simulink model "navigation_filter_flat_earth_noise"  (R2024a)
settings: Solver=VariableStepAuto  StartTime=0.0  StopTime=time(end)  RelTol=1e-3
values from neighbouring files (symbols this model uses):
  pos = pos_f    [test_traj_gen_v2 1.m]    (also in test_traj_gen_v2.m)
  rpy = zeros(length(time),3)    [test_traj_gen_v2 1.m]    (also in test_traj_gen_v2.m)
  ST = 1/100    (= 0.01)    [test_traj_gen_v2 1.m]    (also in test_traj_gen_v2.m)
  vel_n = vel_n_f    [test_traj_gen_v2 1.m]    (also in test_traj_gen_v2.m)
undefined symbols (not defined in the file or in its folder): DiscIntNeverNeededParam
libraries: simulink x8, cstblocks x3
settings Model: Creator=Lorenzo  LastModifiedBy=Lorenzo
settings RTWCC: GPUComputeCapability=3.5

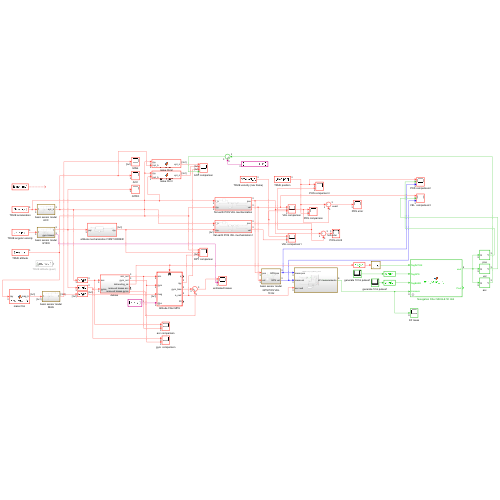
[thumbnail: Simulink's stored preview of the top-level diagram]
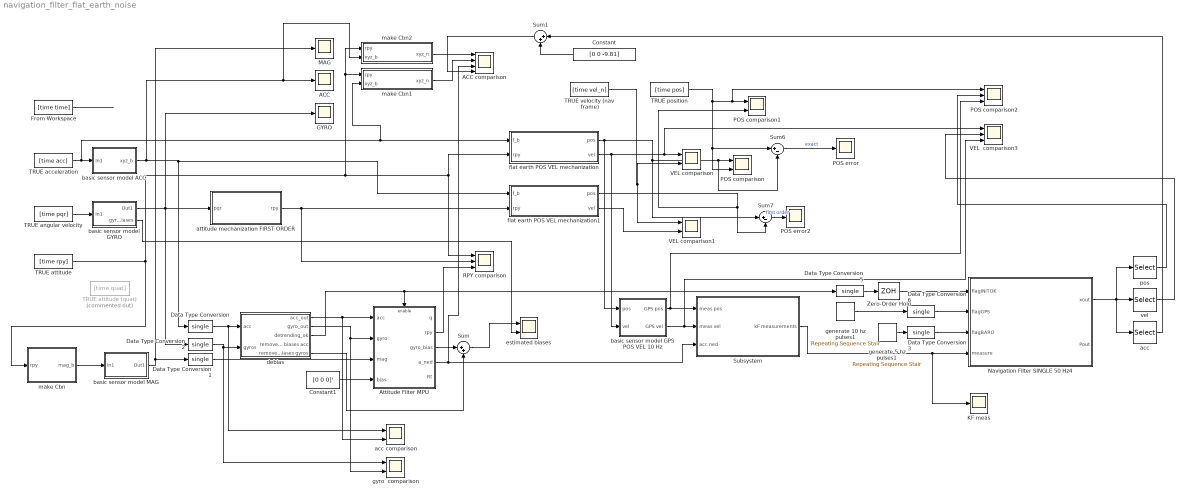
== system navigation_filter_flat_earth_noise ==
  ACC : Scope
  ACC comparison : Scope  NumInputPorts=4
  Attitude Filter MPU : Subsystem  mask{T=ST}
      mask prompts: T "Sample Time"
  Constant : Constant  Value=[0 0 -9.81]
  Constant1 : Constant  Value=[0 0 0]'  OutDataTypeStr=single
  Data Type Conversion{,1..3,5..6} (6 alike) : DataTypeConversion  OutDataTypeStr=single  SaturateOnIntegerOverflow=off  RndMeth=Floor
  From Workspace : FromWorkspace  VariableName=[time time]  SampleTime=ST
  GYRO : Scope
  KF meas : Scope
  MAG : Scope
  "Navigation Filter SINGLE 50 Hz4 " : MATLAB Function  TreatAsAtomicUnit=on  mask{Q=single(diag([1e-8, 1e-4, 1e-2, 1e-8, 1e-4, 1e-2, 1e-5, 1e-4, 0.010]))*2, GPS_cov=single([0.1, 0.1, 10, 10, 0.36])/2, IMU_cov=single([15*[0.07, 0.07] 10*0.09])/2, BARO_cov=single(1.7)/2}
      mask prompts: Q "Q matrix"; GPS_cov "R matrix - GPS covariance [px py vx vy vz]"; IMU_cov "R matrix - IMU covariance [ax ay az]"; BARO_cov "R matrix - BARO covariance"
  POS comparison : Scope  NumInputPorts=2
  POS comparison1 : Scope  NumInputPorts=2
  POS comparison2 : Scope  NumInputPorts=3
  POS error : Scope
  POS error2 : Scope
  RPY comparison : Scope  NumInputPorts=3
  Subsystem : Subsystem
  Sum : Sum  Inputs=|++
  Sum1 : Sum  Inputs=|++
  Sum6 : Sum  Inputs=|+-
  Sum7 : Sum  Inputs=|+-
  TRUE acceleration : FromWorkspace  VariableName=[time acc]  SampleTime=ST
  TRUE angular velocity : FromWorkspace  VariableName=[time pqr]  SampleTime=ST
  TRUE attitude : FromWorkspace  VariableName=[time rpy]  SampleTime=ST
  TRUE attitude (quat) : FromWorkspace  Commented=on  VariableName=[time quat]
  TRUE position : FromWorkspace  VariableName=[time pos]  SampleTime=ST
  TRUE velocity (nav frame) : FromWorkspace  VariableName=[time vel_n]  SampleTime=ST
  VEL  comparison3 : Scope  NumInputPorts=3
  VEL comparison : Scope  NumInputPorts=2
  VEL comparison1 : Scope  NumInputPorts=2
  Zero-Order Hold : ZeroOrderHold  SampleTime=0.02
  acc : Selector  InputPortWidth=9  IndexOptions=Index vector (dialog)  Indices=[1 4 7]+2  OutputSizes=1
  acc comparison : Scope  NumInputPorts=2
  attitude mechanization FIRST ORDER : Subsystem
  basic sensor model ACC : Subsystem
  basic sensor model GPS POS VEL 10 Hz : Subsystem
  basic sensor model GYRO : Subsystem
  basic sensor model MAG : Subsystem
  "debias " : Subsystem
  estimated biases : Scope  NumInputPorts=2
  flat earth POS VEL mechanization : Subsystem
  flat earth POS VEL mechanization1 : Subsystem
  generate 10 hz pulses1 : simulink/Sources/Repeating Sequence Stair  OutValues=[ 0 0 0 0 1].'  tsamp=1/50  OutMin=[]  OutMax=[]  OutDataTypeStr=double  OutputDataTypeScalingMode=double  OutDataType=fixdt(0,8)  ConRadixGroup=Best Precision: Vector-wise  OutScaling=2^-12
  generate 5 hz pulses1 : simulink/Sources/Repeating Sequence Stair  OutValues=[ 0 0 0 0 0 0 0 0 1].'  tsamp=1/50  OutMin=[]  OutMax=[]  OutDataTypeStr=double  OutputDataTypeScalingMode=double  OutDataType=fixdt(0,8)  ConRadixGroup=Best Precision: Vector-wise  OutScaling=2^-12
  gyro  comparison : Scope  NumInputPorts=2
  make Cbn : MATLAB Function  TreatAsAtomicUnit=on
  make Cbn1 : MATLAB Function  TreatAsAtomicUnit=on
  make Cbn2 : MATLAB Function  TreatAsAtomicUnit=on
  pos : Selector  InputPortWidth=9  IndexOptions=Index vector (dialog)  Indices=[1 4 7]  OutputSizes=1
  vel : Selector  InputPortWidth=9  IndexOptions=Index vector (dialog)  Indices=[1 4 7]+1  OutputSizes=1
  wires:
  From Workspace/1 -> ?
  TRUE position/1 -> POS comparison2/1, POS comparison1/1, Sum6/1, POS comparison/2
  TRUE velocity (nav frame)/1 -> VEL comparison1/1, VEL comparison/2
  flat earth POS VEL mechanization/1(pos) -> basic sensor model GPS POS VEL 10 Hz/1(pos), Sum7/1, Sum6/2, POS comparison/1
  flat earth POS VEL mechanization/2(vel) -> basic sensor model GPS POS VEL 10 Hz/2(vel), VEL  comparison3/1, VEL comparison/1
  TRUE angular velocity/1 -> basic sensor model GYRO/1(In1)
  attitude mechanization FIRST ORDER/1(rpy) -> RPY comparison/2, flat earth POS VEL mechanization1/2(rpy)
  TRUE attitude/1 -> make Cbn/1(rpy), make Cbn1/1(rpy), make Cbn2/1(rpy), RPY comparison/1, flat earth POS VEL mechanization/2(rpy)
  Sum6/1 -> POS error/1  "exact"
  Sum7/1 -> POS error2/1  "first order"
  flat earth POS VEL mechanization1/1(pos) -> Sum7/2, POS comparison1/2
  basic sensor model ACC/1(xyz_b) -> make Cbn2/2(xyz_b), ACC/1, Data Type Conversion/1, flat earth POS VEL mechanization1/1(f_b)
  TRUE acceleration/1 -> make Cbn1/2(xyz_b), flat earth POS VEL mechanization/1(f_b), basic sensor model ACC/1(In1)
  basic sensor model GYRO/1(Out1) -> attitude mechanization FIRST ORDER/1(pqr), Data Type Conversion2/1, GYRO/1
  flat earth POS VEL mechanization1/2(vel) -> VEL comparison1/2
  make Cbn/1(mag_b) -> basic sensor model MAG/1(In1)
  basic sensor model MAG/1(Out1) -> MAG/1, Data Type Conversion1/1
  Constant1/1 -> Attitude Filter MPU/4(bias)
  Attitude Filter MPU/2(rpy) -> RPY comparison/3
  Data Type Conversion/1 -> acc comparison/1, "debias "/1(acc)
  Data Type Conversion2/1 -> gyro  comparison/1, "debias "/2(gyros)
  Attitude Filter MPU/3(gyro_bias) -> Sum/1
  basic sensor model GYRO/2(gyro biases) -> estimated biases/2
  "debias "/3(detrending_ok) -> Attitude Filter MPU/Enable, Data Type Conversion5/1
  "debias "/1(acc_out) -> acc comparison/2, Attitude Filter MPU/1(acc)
  "debias "/2(gyro_out) -> gyro  comparison/2, Attitude Filter MPU/2(gyro)
  Data Type Conversion1/1 -> Attitude Filter MPU/3(mag)
  "debias "/5(removed biases gyros) -> Sum/2
  Sum/1 -> estimated biases/1
  basic sensor model GPS POS VEL 10 Hz/1("GPS pos ") -> POS comparison2/3, Subsystem/1("meas pos ")
  "Navigation Filter SINGLE 50 Hz4 "/1(xout) -> acc/1, vel/1, pos/1
  pos/1 -> POS comparison2/2
  vel/1 -> VEL  comparison3/2
  basic sensor model GPS POS VEL 10 Hz/2(GPS vel) -> VEL  comparison3/3, Subsystem/2(meas vel)
  acc/1 -> Sum1/1
  Attitude Filter MPU/4(a_ned) -> Subsystem/3(acc ned), ACC comparison/3
  Subsystem/1(kF measurements) -> KF meas/1, "Navigation Filter SINGLE 50 Hz4 "/4(measure)
  generate 10 hz pulses1/1 -> Data Type Conversion6/1
  generate 5 hz pulses1/1 -> Data Type Conversion3/1
  Data Type Conversion6/1 -> "Navigation Filter SINGLE 50 Hz4 "/2(flagGPS)
  Data Type Conversion3/1 -> "Navigation Filter SINGLE 50 Hz4 "/3(flagBARO)
  Data Type Conversion5/1 -> Zero-Order Hold/1
  make Cbn1/1(xyz_n) -> ACC comparison/2
  make Cbn2/1(xyz_n) -> ACC comparison/1
  Sum1/1 -> ACC comparison/4
  Constant/1 -> Sum1/2
  Zero-Order Hold/1 -> "Navigation Filter SINGLE 50 Hz4 "/1(flagINITOK)

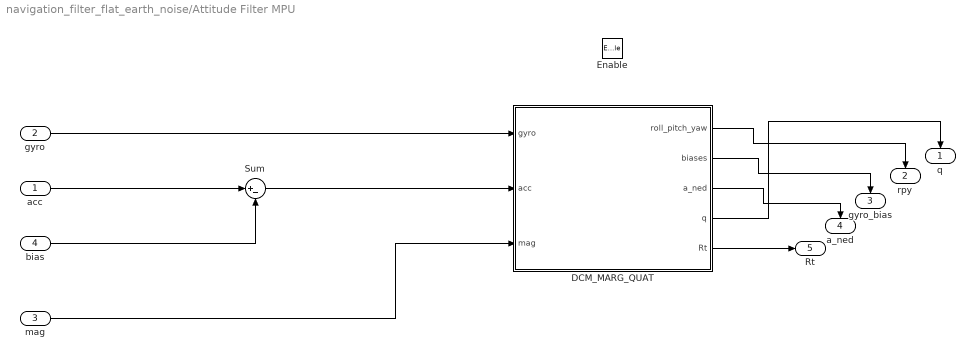
== system navigation_filter_flat_earth_noise/Attitude Filter MPU ==
  acc : Inport
  gyro : Inport  Port=2
  mag : Inport  Port=3
  bias : Inport  Port=4
  Enable : EnablePort  StatesWhenEnabling=reset
  DCM_MARG_QUAT : Subsystem  mask{Kp=0.15, Ki=0.005, tau=40, T=T}
      mask prompts: Kp "Proportional Gain"; Ki "Integral Gain"; tau "Biases Time Constant"; T "Sample Time"
  Sum : Sum  Inputs=|+-
  q : Outport  PortDimensions=4  InitialOutput=[1 0 0 0]'
  rpy : Outport  Port=2  PortDimensions=3  InitialOutput=[0 0 0]'
  gyro_bias : Outport  Port=3  PortDimensions=3  InitialOutput=[0 0 0]'
  a_ned : Outport  Port=4  InitialOutput=[0 0 0]'
  Rt : Outport  Port=5
  wires:
  mag/1 -> DCM_MARG_QUAT/3(mag)
  DCM_MARG_QUAT/4(q) -> q/1
  bias/1 -> Sum/2
  Sum/1 -> DCM_MARG_QUAT/2(acc)
  acc/1 -> Sum/1
  DCM_MARG_QUAT/3(a_ned) -> a_ned/1
  DCM_MARG_QUAT/1(roll_pitch_yaw) -> rpy/1
  gyro/1 -> DCM_MARG_QUAT/1(gyro)
  DCM_MARG_QUAT/2(biases) -> gyro_bias/1
  DCM_MARG_QUAT/5(Rt) -> Rt/1

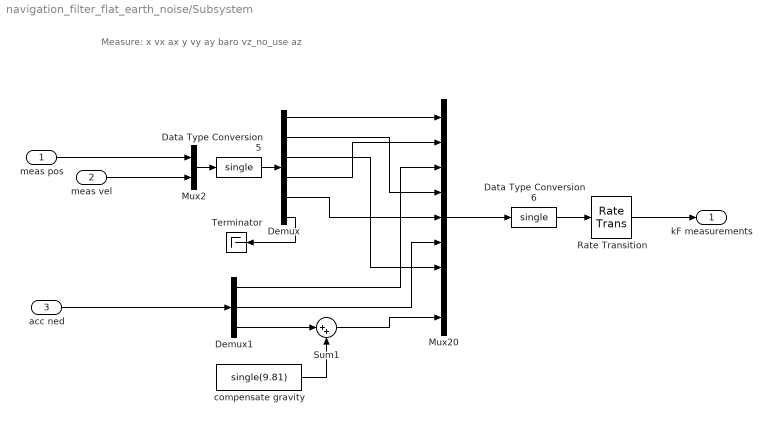
== system navigation_filter_flat_earth_noise/Subsystem ==
  note: Measure: x vx ax y vy ay baro vz_no_use az
  "meas pos " : Inport
  meas vel : Inport  Port=2
  acc ned : Inport  Port=3
  Data Type Conversion5 : DataTypeConversion  OutDataTypeStr=single  SaturateOnIntegerOverflow=off  RndMeth=Floor
  Data Type Conversion6 : DataTypeConversion  OutDataTypeStr=single  SaturateOnIntegerOverflow=off  RndMeth=Floor
  Demux : Demux  Outputs=6
  Demux1 : Demux  Outputs=3
  Mux2 : Mux  Inputs=2
  Mux20 : Mux  Inputs=9
  Rate Transition : RateTransition  OutPortSampleTime=1/50
  Sum1 : Sum  Inputs=|++
  Terminator : Terminator
  compensate gravity : Constant  Value=single(9.81)
  kF measurements : Outport
  wires:
  Demux/5 -> Mux20/5
  Sum1/1 -> Mux20/9
  Demux/4 -> Mux20/2
  Mux20/1 -> Data Type Conversion6/1
  Demux1/3 -> Sum1/1
  Data Type Conversion5/1 -> Demux/1
  Demux/6 -> Terminator/1
  Demux/1 -> Mux20/1
  ? -> Mux20/8
  Data Type Conversion6/1 -> Rate Transition/1
  Mux2/1 -> Data Type Conversion5/1
  Demux1/2 -> Mux20/6
  "meas pos "/1 -> Mux2/1
  compensate gravity/1 -> Sum1/2
  Demux/3 -> Mux20/7
  Demux1/1 -> Mux20/3
  Demux/2 -> Mux20/4
  meas vel/1 -> Mux2/2
  acc ned/1 -> Demux1/1
  Rate Transition/1 -> kF measurements/1

== system navigation_filter_flat_earth_noise/attitude mechanization FIRST ORDER ==
  pqr : Inport
  Attitude Mechanization : MATLAB Function  TreatAsAtomicUnit=on
  rpy_mem : UnitDelay  InitialCondition=rpy(1,:)'  SampleTime=-1  HasFrameUpgradeWarning=on
  rpy : Outport
  wires:
  pqr/1 -> Attitude Mechanization/1(pqr)
  rpy_mem/1 -> Attitude Mechanization/2(rpy_)
  Attitude Mechanization/1(rpy) -> rpy_mem/1, rpy/1

== system navigation_filter_flat_earth_noise/basic sensor model ACC ==
  note: [0.05 0.1 0.15]
  In1 : Inport
  Add : Sum  Inputs=+++
  Mux : Mux  Inputs=2
  Scope : Scope
  White Noise acc : RandomNumber  DisableCoverage=on  Mean=[0 0 0 ]  Variance=[0.006 0.006 0.006].^2  Seed=[1 2 3]  SampleTime=1/50
  bias : Constant  Value=[0.05 0.1 0.15]
  xyz_b : Outport
  wires:
  In1/1 -> Mux/2, Add/1
  White Noise acc/1 -> Add/3
  bias/1 -> Add/2
  Mux/1 -> Scope/1
  Add/1 -> Mux/1, xyz_b/1

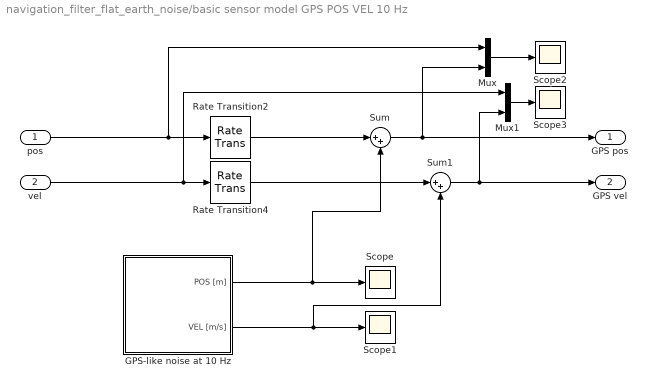
== system navigation_filter_flat_earth_noise/basic sensor model GPS POS VEL 10 Hz ==
  pos : Inport
  vel : Inport  Port=2
  GPS-like noise at 10 Hz : Subsystem  mask{AMPX=3, AMPY=3, AMPZ=0.5, newnoise=off, seed_user=0}
      mask prompts: AMPX "gps approx max error X [m]"; AMPY "gps approx max error Y [m]"; AMPZ "gps approx max error Z [m]"; newnoise "new noise at each run"; seed_user "user provided seed value"
      mask init:
      | if newnoise,
      |         seedx=rand(1)*1000;
      |         seedy=rand(1)*1000;
      |         seedz=rand(1)*1000;
      |     else
      |         seedx=seed_user;
      |         seedy=seed_user+1;
      |         seedz=seed_user+2;
      |     end
      mask DialogControl ParameterGroupVar Prompt: Noise generation
  Mux : Mux  Inputs=2
  Mux1 : Mux  Inputs=2
  Rate Transition2 : RateTransition  OutPortSampleTime=1/10
  Rate Transition4 : RateTransition  OutPortSampleTime=1/10
  Scope{,1..3} (4 alike) : Scope
  Sum : Sum  Inputs=|++
  Sum1 : Sum  Inputs=|++
  "GPS pos " : Outport
  GPS vel : Outport  Port=2
  wires:
  pos/1 -> Mux/1, Rate Transition2/1
  vel/1 -> Mux1/1, Rate Transition4/1
  GPS-like noise at 10 Hz/2(VEL [m/s]) -> Sum1/2, Scope1/1
  GPS-like noise at 10 Hz/1(POS [m]) -> Sum/2, Scope/1
  Mux/1 -> Scope2/1
  Sum/1 -> "GPS pos "/1, Mux/2
  Sum1/1 -> Mux1/2, GPS vel/1
  Rate Transition2/1 -> Sum/1
  Rate Transition4/1 -> Sum1/1
  Mux1/1 -> Scope3/1

== system navigation_filter_flat_earth_noise/basic sensor model GYRO ==
  In1 : Inport
  Add : Sum  Inputs=+++
  Mux : Mux  Inputs=2
  Scope : Scope
  White Noise gyro : RandomNumber  DisableCoverage=on  Mean=[0 0 0]  Variance=[0.003 0.003 0.003].^2  Seed=[4 5 6]  SampleTime=1/50
  bias : Constant  Value=[0.03 0.06 0.09]
  Out1 : Outport
  gyro biases : Outport  Port=2
  wires:
  White Noise gyro/1 -> Add/3
  bias/1 -> Add/2, gyro biases/1
  Mux/1 -> Scope/1
  In1/1 -> Mux/2, Add/1
  Add/1 -> Mux/1, Out1/1

== system navigation_filter_flat_earth_noise/basic sensor model MAG ==
  In1 : Inport
  Add : Sum  Inputs=+++
  Mux : Mux  Inputs=2
  Scope : Scope
  White Noise mag : RandomNumber  DisableCoverage=on  Mean=[0 0 0]  Variance=[0.003 0.003 0.003].^2  Seed=[7 8 9]  SampleTime=1/50
  bias : Constant  Value=[0.0 0.0 0.0]
  Out1 : Outport
  wires:
  Add/1 -> Out1/1, Mux/1
  In1/1 -> Add/1, Mux/2
  Mux/1 -> Scope/1
  bias/1 -> Add/2
  White Noise mag/1 -> Add/3

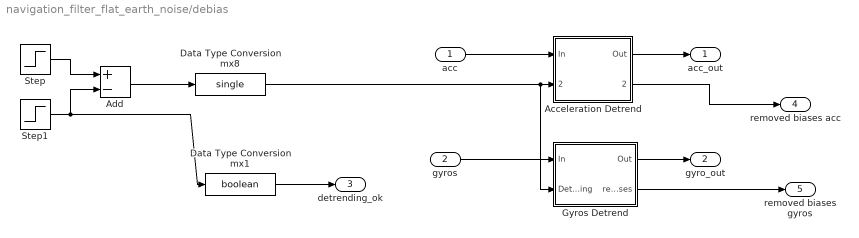
== system navigation_filter_flat_earth_noise/debias  ==
  acc : Inport
  gyros : Inport  Port=2
  "Acceleration Detrend " : Subsystem  mask{ST2=ST}
      mask prompts: ST2 "Sample Time"
  Add : Sum  Inputs=+-
  Data Type Conversion mx1 : DataTypeConversion  OutDataTypeStr=boolean  RndMeth=Round
  Data Type Conversion mx8 : DataTypeConversion  OutDataTypeStr=single  RndMeth=Round
  Gyros Detrend : Subsystem  mask{ST2=ST}
      mask prompts: ST2 "Sample Time"
  Step : Step  Time=0.1  SampleTime=ST
  Step1 : Step  SampleTime=ST
  acc_out : Outport
  gyro_out : Outport  Port=2
  detrending_ok : Outport  Port=3
  removed biases acc : Outport  Port=4
  removed biases gyros : Outport  Port=5
  wires:
  Step/1 -> Add/1
  Step1/1 -> Add/2, Data Type Conversion mx1/1
  Add/1 -> Data Type Conversion mx8/1
  acc/1 -> "Acceleration Detrend "/1(In)
  gyros/1 -> Gyros Detrend/1(In)
  "Acceleration Detrend "/1(Out) -> acc_out/1
  Gyros Detrend/1(Out) -> gyro_out/1
  Data Type Conversion mx1/1 -> detrending_ok/1
  Data Type Conversion mx8/1 -> Gyros Detrend/2(Detrending), "Acceleration Detrend "/2(Detrending)
  "Acceleration Detrend "/2(removed biases) -> removed biases acc/1
  Gyros Detrend/2(removed biases) -> removed biases gyros/1

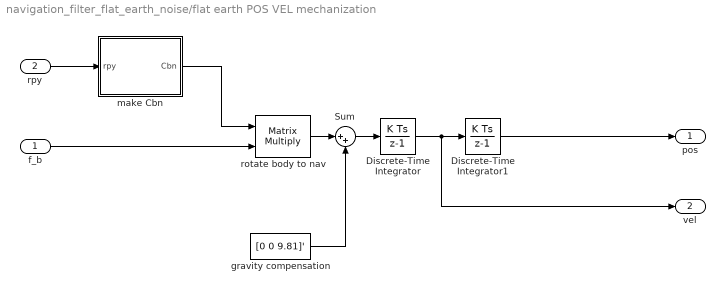
== system navigation_filter_flat_earth_noise/flat earth POS VEL mechanization ==
  f_b : Inport
  rpy : Inport  Port=2
  Discrete-Time Integrator : DiscreteIntegrator  InitialCondition=vel_n(1,:)  SampleTime=-1  ICPrevOutput=DiscIntNeverNeededParam  ICPrevScaledInput=DiscIntNeverNeededParam
  Discrete-Time Integrator1 : DiscreteIntegrator  InitialCondition=pos(1,:)  SampleTime=-1  ICPrevOutput=DiscIntNeverNeededParam  ICPrevScaledInput=DiscIntNeverNeededParam
  Sum : Sum  Inputs=|++
  gravity compensation : Constant  Value=[0 0 9.81]'
  make Cbn : MATLAB Function  TreatAsAtomicUnit=on
  rotate body to nav : Product  Multiplication=Matrix(*)
  pos : Outport
  vel : Outport  Port=2
  wires:
  rotate body to nav/1 -> Sum/1
  gravity compensation/1 -> Sum/2
  Discrete-Time Integrator/1 -> vel/1, Discrete-Time Integrator1/1
  make Cbn/1(Cbn) -> rotate body to nav/1
  Discrete-Time Integrator1/1 -> pos/1
  Sum/1 -> Discrete-Time Integrator/1
  f_b/1 -> rotate body to nav/2
  rpy/1 -> make Cbn/1(rpy)

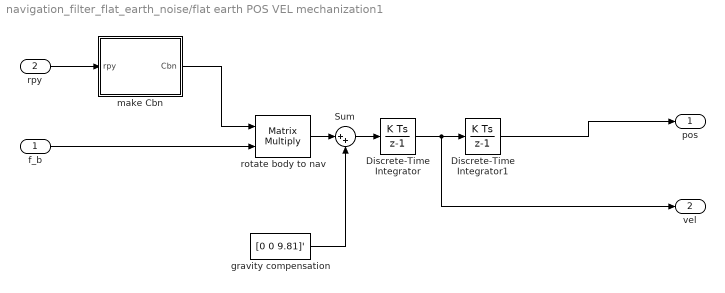
== system navigation_filter_flat_earth_noise/flat earth POS VEL mechanization1 ==
  f_b : Inport
  rpy : Inport  Port=2
  Discrete-Time Integrator : DiscreteIntegrator  InitialCondition=vel_n(1,:)  SampleTime=-1  ICPrevOutput=DiscIntNeverNeededParam  ICPrevScaledInput=DiscIntNeverNeededParam
  Discrete-Time Integrator1 : DiscreteIntegrator  InitialCondition=pos(1,:)  SampleTime=-1  ICPrevOutput=DiscIntNeverNeededParam  ICPrevScaledInput=DiscIntNeverNeededParam
  Sum : Sum  Inputs=|++
  gravity compensation : Constant  Value=[0 0 9.81]'
  make Cbn : MATLAB Function  TreatAsAtomicUnit=on
  rotate body to nav : Product  Multiplication=Matrix(*)
  pos : Outport
  vel : Outport  Port=2
  wires:
  rpy/1 -> make Cbn/1(rpy)
  f_b/1 -> rotate body to nav/2
  Sum/1 -> Discrete-Time Integrator/1
  Discrete-Time Integrator1/1 -> pos/1
  make Cbn/1(Cbn) -> rotate body to nav/1
  Discrete-Time Integrator/1 -> Discrete-Time Integrator1/1, vel/1
  gravity compensation/1 -> Sum/2
  rotate body to nav/1 -> Sum/1

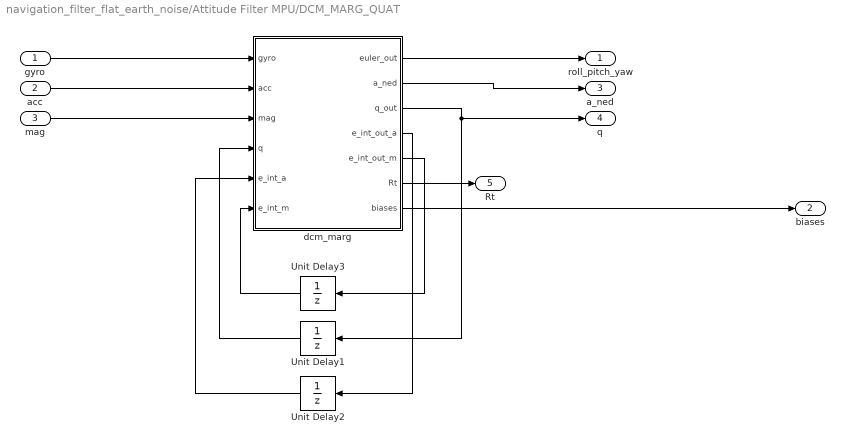
== system navigation_filter_flat_earth_noise/Attitude Filter MPU/DCM_MARG_QUAT ==
  gyro : Inport
  acc : Inport  Port=2
  mag : Inport  Port=3
  Unit Delay1 : UnitDelay  InitialCondition=[1;0;0;0]  SampleTime=T  HasFrameUpgradeWarning=on
  Unit Delay2 : UnitDelay  SampleTime=T  HasFrameUpgradeWarning=on
  Unit Delay3 : UnitDelay  SampleTime=T  HasFrameUpgradeWarning=on
  dcm_marg : MATLAB Function  TreatAsAtomicUnit=on
  roll_pitch_yaw : Outport
  biases : Outport  Port=2
  a_ned : Outport  Port=3
  q : Outport  Port=4
  Rt : Outport  Port=5
  wires:
  Unit Delay3/1 -> dcm_marg/6(e_int_m)
  dcm_marg/5(e_int_out_m) -> Unit Delay3/1
  dcm_marg/2(a_ned) -> a_ned/1
  dcm_marg/1(euler_out) -> roll_pitch_yaw/1
  gyro/1 -> dcm_marg/1(gyro)
  acc/1 -> dcm_marg/2(acc)
  mag/1 -> dcm_marg/3(mag)
  dcm_marg/3(q_out) -> q/1, Unit Delay1/1
  Unit Delay1/1 -> dcm_marg/4(q)
  dcm_marg/4(e_int_out_a) -> Unit Delay2/1
  Unit Delay2/1 -> dcm_marg/5(e_int_a)
  dcm_marg/7(biases) -> biases/1
  dcm_marg/6(Rt) -> Rt/1

== system navigation_filter_flat_earth_noise/basic sensor model GPS POS VEL 10 Hz/GPS-like noise at 10 Hz ==
  GPS-like noise X : Subsystem
  GPS-like noise Y : Subsystem
  GPS-like noise Z : Subsystem
  Mux : Mux  Inputs=3
  Mux1 : Mux  Inputs=3
  POS [m] : Outport
  VEL [m/s] : Outport  Port=2
  wires:
  GPS-like noise Y/1(pos) -> Mux/2
  Mux/1 -> POS [m]/1
  GPS-like noise X/1(pos) -> Mux/1
  GPS-like noise Z/2(vel) -> Mux1/3
  GPS-like noise Y/2(vel) -> Mux1/2
  GPS-like noise Z/1(pos) -> Mux/3
  GPS-like noise X/2(vel) -> Mux1/1
  Mux1/1 -> VEL [m/s]/1

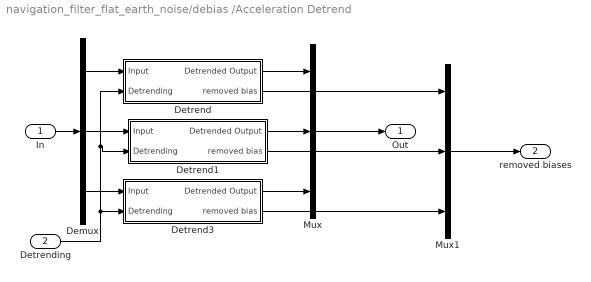
== system navigation_filter_flat_earth_noise/debias /Acceleration Detrend  ==
  In : Inport
  Detrending : Inport  Port=2
  Demux : Demux  Outputs=3
      settings: DisplayOption=none
  Detrend : Subsystem  mask{ST=ST2}
      mask prompts: ST "Sample Time"
  Detrend1 : Subsystem  mask{ST=ST2}
      mask prompts: ST "Sample Time"
  Detrend3 : Subsystem  mask{ST=ST2}
      mask prompts: ST "Sample Time"
  Mux : Mux  Inputs=3
  Mux1 : Mux  Inputs=3
  Out : Outport
  removed biases : Outport  Port=2
  wires:
  Detrending/1 -> Detrend3/2(Detrending), Detrend1/2(Detrending), Detrend/2(Detrending)
  Demux/3 -> Detrend3/1(Input)
  In/1 -> Demux/1
  Demux/2 -> Detrend1/1(Input)
  Demux/1 -> Detrend/1(Input)
  Mux/1 -> Out/1
  Detrend3/1(Detrended Output) -> Mux/3
  Detrend1/1(Detrended Output) -> Mux/2
  Detrend/1(Detrended Output) -> Mux/1
  Mux1/1 -> removed biases/1
  Detrend/2("removed bias ") -> Mux1/1
  Detrend1/2("removed bias ") -> Mux1/2
  Detrend3/2(removed bias) -> Mux1/3

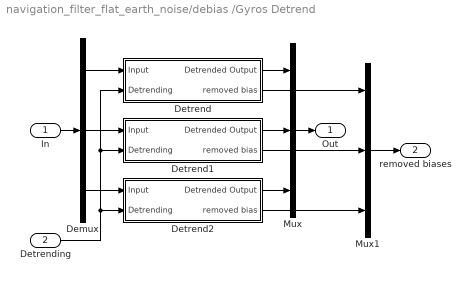
== system navigation_filter_flat_earth_noise/debias /Gyros Detrend ==
  In : Inport
  Detrending : Inport  Port=2
  Demux : Demux  Outputs=3
      settings: DisplayOption=none
  Detrend : Subsystem  mask{ST=ST2}
      mask prompts: ST "Sample Time"
  Detrend1 : Subsystem  mask{ST=ST2}
      mask prompts: ST "Sample Time"
  Detrend2 : Subsystem  mask{ST=ST2}
      mask prompts: ST "Sample Time"
  Mux : Mux  Inputs=3
  Mux1 : Mux  Inputs=3
  Out : Outport
  removed biases : Outport  Port=2
  wires:
  Detrend/1(Detrended Output) -> Mux/1
  Detrend1/1(Detrended Output) -> Mux/2
  Mux/1 -> Out/1
  Demux/1 -> Detrend/1(Input)
  Demux/2 -> Detrend1/1(Input)
  In/1 -> Demux/1
  Demux/3 -> Detrend2/1(Input)
  Detrending/1 -> Detrend2/2(Detrending), Detrend1/2(Detrending), Detrend/2(Detrending)
  Detrend2/1(Detrended Output) -> Mux/3
  Mux1/1 -> removed biases/1
  Detrend1/2(removed bias) -> Mux1/2
  Detrend/2(removed bias) -> Mux1/1
  Detrend2/2(removed bias) -> Mux1/3

== system navigation_filter_flat_earth_noise/basic sensor model GPS POS VEL 10 Hz/GPS-like noise at 10 Hz/GPS-like noise X ==
  Discrete-Time Integrator : DiscreteIntegrator  SampleTime=1/10  ICPrevOutput=DiscIntNeverNeededParam  ICPrevScaledInput=DiscIntNeverNeededParam
  Gain : Gain  Gain=0.75
  Gain1 : Gain  Gain=AMPX
  LTI System1 : cstblocks/LTI System  sys=c2d(tf(1,[0.75 1])*tf([3000 0],[3000 1]),1/10)  IC=[]  PadeOrder=0
  Random Number : RandomNumber  Variance=0.01  Seed=seedx  SampleTime=1/10
  pos : Outport
  vel : Outport  Port=2
  wires:
  Discrete-Time Integrator/1 -> pos/1
  LTI System1/1 -> vel/1, Discrete-Time Integrator/1
  Random Number/1 -> Gain1/1
  Gain/1 -> LTI System1/1
  Gain1/1 -> Gain/1

== system navigation_filter_flat_earth_noise/basic sensor model GPS POS VEL 10 Hz/GPS-like noise at 10 Hz/GPS-like noise Y ==
  Discrete-Time Integrator : DiscreteIntegrator  SampleTime=1/10  ICPrevOutput=DiscIntNeverNeededParam  ICPrevScaledInput=DiscIntNeverNeededParam
  Gain : Gain  Gain=0.75
  Gain1 : Gain  Gain=AMPY
  LTI System1 : cstblocks/LTI System  sys=c2d(tf(1,[0.75 1])*tf([3000 0],[3000 1]),1/10)  IC=[]  PadeOrder=0
  Random Number : RandomNumber  Variance=0.01  Seed=seedy  SampleTime=1/10
  pos : Outport
  vel : Outport  Port=2
  wires:
  Gain1/1 -> Gain/1
  Gain/1 -> LTI System1/1
  Random Number/1 -> Gain1/1
  LTI System1/1 -> vel/1, Discrete-Time Integrator/1
  Discrete-Time Integrator/1 -> pos/1

== system navigation_filter_flat_earth_noise/basic sensor model GPS POS VEL 10 Hz/GPS-like noise at 10 Hz/GPS-like noise Z ==
  Discrete-Time Integrator : DiscreteIntegrator  SampleTime=1/10  ICPrevOutput=DiscIntNeverNeededParam  ICPrevScaledInput=DiscIntNeverNeededParam
  Gain : Gain  Gain=0.75
  Gain1 : Gain  Gain=AMPZ
  LTI System1 : cstblocks/LTI System  sys=c2d(tf(1,[0.75 1])*tf([3000 0],[3000 1]),1/10)  IC=[]  PadeOrder=0
  Random Number : RandomNumber  Variance=0.01  Seed=seedz  SampleTime=1/10
  pos : Outport
  vel : Outport  Port=2
  wires:
  Discrete-Time Integrator/1 -> pos/1
  LTI System1/1 -> vel/1, Discrete-Time Integrator/1
  Random Number/1 -> Gain1/1
  Gain/1 -> LTI System1/1
  Gain1/1 -> Gain/1

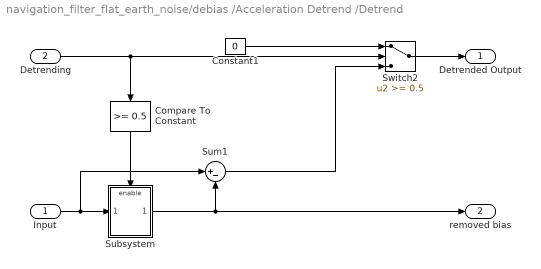
== system navigation_filter_flat_earth_noise/debias /Acceleration Detrend /Detrend ==
  Input : Inport
  Detrending : Inport  Port=2
  Compare To Constant : simulink/Logic and Bit Operations/Compare To Constant  relop=>=  const=0.5  OutDataTypeStr=boolean
  Constant1 : Constant  Value=0  OutDataTypeStr=single
  Subsystem : Subsystem  TreatAsAtomicUnit=on
  Sum1 : Sum  Inputs=|+-  InputSameDT=on  SaturateOnIntegerOverflow=on  OutDataTypeStr=Inherit: Same as first input
  Switch2 : Switch  Threshold=0.5
  Detrended Output : Outport
  "removed bias " : Outport  Port=2
  wires:
  Switch2/1 -> Detrended Output/1
  Detrending/1 -> Switch2/2, Compare To Constant/1
  Constant1/1 -> Switch2/1
  Input/1 -> Sum1/1, Subsystem/1(In1)
  Sum1/1 -> Switch2/3
  Compare To Constant/1 -> Subsystem/Enable
  Subsystem/1("removed bias ") -> "removed bias "/1, Sum1/2

== system navigation_filter_flat_earth_noise/debias /Acceleration Detrend /Detrend1 ==
  Input : Inport
  Detrending : Inport  Port=2
  Compare To Constant : simulink/Logic and Bit Operations/Compare To Constant  relop=>=  const=0.5  OutDataTypeStr=boolean
  Constant1 : Constant  Value=0  OutDataTypeStr=single
  Subsystem : Subsystem  TreatAsAtomicUnit=on
  Sum1 : Sum  Inputs=|+-  InputSameDT=on  SaturateOnIntegerOverflow=on  OutDataTypeStr=Inherit: Same as first input
  Switch2 : Switch  Threshold=0.5
  Detrended Output : Outport
  "removed bias " : Outport  Port=2
  wires:
  Subsystem/1("removed bias ") -> "removed bias "/1, Sum1/2
  Compare To Constant/1 -> Subsystem/Enable
  Sum1/1 -> Switch2/3
  Input/1 -> Subsystem/1(In1), Sum1/1
  Constant1/1 -> Switch2/1
  Detrending/1 -> Compare To Constant/1, Switch2/2
  Switch2/1 -> Detrended Output/1

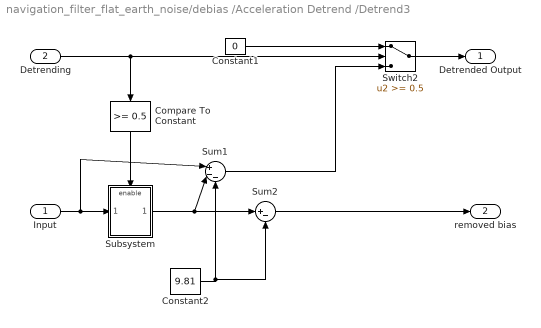
== system navigation_filter_flat_earth_noise/debias /Acceleration Detrend /Detrend3 ==
  Input : Inport
  Detrending : Inport  Port=2
  Compare To Constant : simulink/Logic and Bit Operations/Compare To Constant  relop=>=  const=0.5  OutDataTypeStr=boolean
  Constant1 : Constant  Value=0  OutDataTypeStr=single
  Constant2 : Constant  Value=9.81  OutDataTypeStr=single
  Subsystem : Subsystem  TreatAsAtomicUnit=on
  Sum1 : Sum  Inputs=|+--  InputSameDT=on  SaturateOnIntegerOverflow=on  OutDataTypeStr=Inherit: Same as first input
  Sum2 : Sum  Inputs=|+-  InputSameDT=on  SaturateOnIntegerOverflow=on  OutDataTypeStr=Inherit: Same as first input
  Switch2 : Switch  Threshold=0.5
  Detrended Output : Outport
  removed bias : Outport  Port=2
  wires:
  Switch2/1 -> Detrended Output/1
  Detrending/1 -> Switch2/2, Compare To Constant/1
  Constant1/1 -> Switch2/1
  Input/1 -> Sum1/1, Subsystem/1(In1)
  Sum1/1 -> Switch2/3
  Compare To Constant/1 -> Subsystem/Enable
  Constant2/1 -> Sum2/2, Sum1/3
  Subsystem/1(Out2) -> Sum2/1, Sum1/2
  Sum2/1 -> removed bias/1

== system navigation_filter_flat_earth_noise/debias /Gyros Detrend/Detrend ==
  Input : Inport
  Detrending : Inport  Port=2
  Compare To Constant : simulink/Logic and Bit Operations/Compare To Constant  relop=>=  const=0.5  OutDataTypeStr=boolean
  Constant1 : Constant  Value=0  OutDataTypeStr=single
  Subsystem : Subsystem  TreatAsAtomicUnit=on
  Sum1 : Sum  Inputs=|+-  InputSameDT=on  SaturateOnIntegerOverflow=on  OutDataTypeStr=Inherit: Same as first input
  Switch2 : Switch  Threshold=0.5
  Detrended Output : Outport
  removed bias : Outport  Port=2
  wires:
  Switch2/1 -> Detrended Output/1
  Detrending/1 -> Switch2/2, Compare To Constant/1
  Constant1/1 -> Switch2/1
  Input/1 -> Sum1/1, Subsystem/1(In1)
  Sum1/1 -> Switch2/3
  Compare To Constant/1 -> Subsystem/Enable
  Subsystem/1(removed bias) -> removed bias/1, Sum1/2

== system navigation_filter_flat_earth_noise/debias /Gyros Detrend/Detrend1 ==
  Input : Inport
  Detrending : Inport  Port=2
  Compare To Constant : simulink/Logic and Bit Operations/Compare To Constant  relop=>=  const=0.5  OutDataTypeStr=boolean
  Constant1 : Constant  Value=0  OutDataTypeStr=single
  Subsystem : Subsystem  TreatAsAtomicUnit=on
  Sum1 : Sum  Inputs=|+-  InputSameDT=on  SaturateOnIntegerOverflow=on  OutDataTypeStr=Inherit: Same as first input
  Switch2 : Switch  Threshold=0.5
  Detrended Output : Outport
  removed bias : Outport  Port=2
  wires:
  Subsystem/1(removed bias) -> removed bias/1, Sum1/2
  Compare To Constant/1 -> Subsystem/Enable
  Sum1/1 -> Switch2/3
  Input/1 -> Subsystem/1(In1), Sum1/1
  Constant1/1 -> Switch2/1
  Detrending/1 -> Compare To Constant/1, Switch2/2
  Switch2/1 -> Detrended Output/1

== system navigation_filter_flat_earth_noise/debias /Gyros Detrend/Detrend2 ==
  Input : Inport
  Detrending : Inport  Port=2
  Compare To Constant : simulink/Logic and Bit Operations/Compare To Constant  relop=>=  const=0.5  OutDataTypeStr=boolean
  Constant1 : Constant  Value=0  OutDataTypeStr=single
  Subsystem : Subsystem  TreatAsAtomicUnit=on
  Sum1 : Sum  Inputs=|+-  InputSameDT=on  SaturateOnIntegerOverflow=on  OutDataTypeStr=Inherit: Same as first input
  Switch2 : Switch  Threshold=0.5
  Detrended Output : Outport
  removed bias : Outport  Port=2
  wires:
  Switch2/1 -> Detrended Output/1
  Detrending/1 -> Switch2/2, Compare To Constant/1
  Constant1/1 -> Switch2/1
  Input/1 -> Sum1/1, Subsystem/1(In1)
  Sum1/1 -> Switch2/3
  Compare To Constant/1 -> Subsystem/Enable
  Subsystem/1(removed bias) -> removed bias/1, Sum1/2

== system navigation_filter_flat_earth_noise/debias /Acceleration Detrend /Detrend/Subsystem ==
  In1 : Inport
  Enable : EnablePort
  Constant : Constant  OutDataTypeStr=single
  Discrete-Time Integrator : DiscreteIntegrator  SampleTime=ST  ICPrevOutput=DiscIntNeverNeededParam  ICPrevScaledInput=DiscIntNeverNeededParam
  Discrete-Time Integrator1 : DiscreteIntegrator  InitialCondition=eps  SampleTime=ST  ICPrevOutput=DiscIntNeverNeededParam  ICPrevScaledInput=DiscIntNeverNeededParam
  Product1 : Product  Inputs=*/  InputSameDT=on  RndMeth=Zero  SaturateOnIntegerOverflow=on  OutDataTypeStr=Inherit: Same as first input
  "removed bias " : Outport
  wires:
  Constant/1 -> Discrete-Time Integrator1/1
  Discrete-Time Integrator1/1 -> Product1/2
  Product1/1 -> "removed bias "/1
  Discrete-Time Integrator/1 -> Product1/1
  In1/1 -> Discrete-Time Integrator/1

== system navigation_filter_flat_earth_noise/debias /Acceleration Detrend /Detrend1/Subsystem ==
  In1 : Inport
  Enable : EnablePort
  Constant : Constant  OutDataTypeStr=single
  Discrete-Time Integrator : DiscreteIntegrator  SampleTime=ST  ICPrevOutput=DiscIntNeverNeededParam  ICPrevScaledInput=DiscIntNeverNeededParam
  Discrete-Time Integrator1 : DiscreteIntegrator  InitialCondition=eps  SampleTime=ST  ICPrevOutput=DiscIntNeverNeededParam  ICPrevScaledInput=DiscIntNeverNeededParam
  Product1 : Product  Inputs=*/  InputSameDT=on  RndMeth=Zero  SaturateOnIntegerOverflow=on  OutDataTypeStr=Inherit: Same as first input
  "removed bias " : Outport
  wires:
  In1/1 -> Discrete-Time Integrator/1
  Discrete-Time Integrator/1 -> Product1/1
  Product1/1 -> "removed bias "/1
  Discrete-Time Integrator1/1 -> Product1/2
  Constant/1 -> Discrete-Time Integrator1/1

== system navigation_filter_flat_earth_noise/debias /Acceleration Detrend /Detrend3/Subsystem ==
  In1 : Inport
  Enable : EnablePort
  Constant : Constant  OutDataTypeStr=single
  Discrete-Time Integrator : DiscreteIntegrator  SampleTime=ST  ICPrevOutput=DiscIntNeverNeededParam  ICPrevScaledInput=DiscIntNeverNeededParam
  Discrete-Time Integrator1 : DiscreteIntegrator  InitialCondition=eps  SampleTime=ST  ICPrevOutput=DiscIntNeverNeededParam  ICPrevScaledInput=DiscIntNeverNeededParam
  Product1 : Product  Inputs=*/  InputSameDT=on  RndMeth=Zero  SaturateOnIntegerOverflow=on  OutDataTypeStr=Inherit: Same as first input
  Out2 : Outport
  wires:
  Constant/1 -> Discrete-Time Integrator1/1
  Discrete-Time Integrator1/1 -> Product1/2
  Product1/1 -> Out2/1
  Discrete-Time Integrator/1 -> Product1/1
  In1/1 -> Discrete-Time Integrator/1

== system navigation_filter_flat_earth_noise/debias /Gyros Detrend/Detrend/Subsystem ==
  In1 : Inport
  Enable : EnablePort
  Constant : Constant  OutDataTypeStr=single
  Discrete-Time Integrator : DiscreteIntegrator  SampleTime=ST  ICPrevOutput=DiscIntNeverNeededParam  ICPrevScaledInput=DiscIntNeverNeededParam
  Discrete-Time Integrator1 : DiscreteIntegrator  InitialCondition=eps  SampleTime=ST  ICPrevOutput=DiscIntNeverNeededParam  ICPrevScaledInput=DiscIntNeverNeededParam
  Product1 : Product  Inputs=*/  InputSameDT=on  RndMeth=Zero  SaturateOnIntegerOverflow=on  OutDataTypeStr=Inherit: Same as first input
  removed bias : Outport
  wires:
  Constant/1 -> Discrete-Time Integrator1/1
  Discrete-Time Integrator1/1 -> Product1/2
  Product1/1 -> removed bias/1
  Discrete-Time Integrator/1 -> Product1/1
  In1/1 -> Discrete-Time Integrator/1

== system navigation_filter_flat_earth_noise/debias /Gyros Detrend/Detrend1/Subsystem ==
  In1 : Inport
  Enable : EnablePort
  Constant : Constant  OutDataTypeStr=single
  Discrete-Time Integrator : DiscreteIntegrator  SampleTime=ST  ICPrevOutput=DiscIntNeverNeededParam  ICPrevScaledInput=DiscIntNeverNeededParam
  Discrete-Time Integrator1 : DiscreteIntegrator  InitialCondition=eps  SampleTime=ST  ICPrevOutput=DiscIntNeverNeededParam  ICPrevScaledInput=DiscIntNeverNeededParam
  Product1 : Product  Inputs=*/  InputSameDT=on  RndMeth=Zero  SaturateOnIntegerOverflow=on  OutDataTypeStr=Inherit: Same as first input
  removed bias : Outport
  wires:
  In1/1 -> Discrete-Time Integrator/1
  Discrete-Time Integrator/1 -> Product1/1
  Product1/1 -> removed bias/1
  Discrete-Time Integrator1/1 -> Product1/2
  Constant/1 -> Discrete-Time Integrator1/1

== system navigation_filter_flat_earth_noise/debias /Gyros Detrend/Detrend2/Subsystem ==
  In1 : Inport
  Enable : EnablePort
  Constant : Constant  OutDataTypeStr=single
  Discrete-Time Integrator : DiscreteIntegrator  SampleTime=ST  ICPrevOutput=DiscIntNeverNeededParam  ICPrevScaledInput=DiscIntNeverNeededParam
  Discrete-Time Integrator1 : DiscreteIntegrator  InitialCondition=eps  SampleTime=ST  ICPrevOutput=DiscIntNeverNeededParam  ICPrevScaledInput=DiscIntNeverNeededParam
  Product1 : Product  Inputs=*/  InputSameDT=on  RndMeth=Zero  SaturateOnIntegerOverflow=on  OutDataTypeStr=Inherit: Same as first input
  removed bias : Outport
  wires:
  Constant/1 -> Discrete-Time Integrator1/1
  Discrete-Time Integrator1/1 -> Product1/2
  Product1/1 -> removed bias/1
  Discrete-Time Integrator/1 -> Product1/1
  In1/1 -> Discrete-Time Integrator/1

== matlab function navigation_filter_flat_earth_noise/flat earth POS VEL mechanization1/make Cbn ==
  data: rpy input; Cbn output
function Cbn = make_Cbn(rpy)
%input:angular velocity at current timestep, latest estimation of attitude
%output> rpy and Cbn


%compute Cbn
Cz=[cos(rpy(3))     sin(rpy(3))     0; ...
    -sin(rpy(3))    cos(rpy(3))     0; ...
    0               0               1];

Cy=[cos(rpy(2))     0               -sin(rpy(2)); ...
    0               1               0; ...
    sin(rpy(2))     0               cos(rpy(2))];

Cx=[1               0               0;...
    0               cos(rpy(1))     sin(rpy(1)); ...
    0               -sin(rpy(1))    cos(rpy(1))];

Cbn = (Cx*Cy*Cz)';

== matlab function navigation_filter_flat_earth_noise/attitude mechanization FIRST ORDER/Attitude Mechanization ==
  data: pqr input; rpy output; rpy_ input; ST parameter size=1
function rpy = attitude_mech(pqr,rpy_,ST)
%input:angular velocity at current timestep, latest estimation of attitude
%output> rpy and Cbn

phi = rpy_(1); 
theta = rpy_(2); 
%create Jacobian that transforms angular rates into rates of Euler
%angles
J = [1, sin(phi)*tan(theta), cos(phi)*tan(theta);
     0, cos(phi),            -sin(phi);
     0, sin(phi)/cos(theta), cos(phi)/cos(theta)];

%integrate
delta_rpy = J*pqr*ST;

rpy=rpy_ + delta_rpy;

== matlab function navigation_filter_flat_earth_noise/make Cbn1 ==
  data: rpy input; xyz_n output; xyz_b input
function xyz_n = rot_to_nav(rpy,xyz_b)

%compute Cbn
Cz=[cos(rpy(3))     sin(rpy(3))     0; ...
    -sin(rpy(3))    cos(rpy(3))     0; ...
    0               0               1];

Cy=[cos(rpy(2))     0               -sin(rpy(2)); ...
    0               1               0; ...
    sin(rpy(2))     0               cos(rpy(2))];

Cx=[1               0               0;...
    0               cos(rpy(1))     sin(rpy(1)); ...
    0               -sin(rpy(1))    cos(rpy(1))];

Cbn = (Cx*Cy*Cz)';
xyz_n = Cbn*xyz_b;

== matlab function navigation_filter_flat_earth_noise/make Cbn ==
  data: rpy input; mag_b output
function mag_b = sim_mag_body(rpy)

% define magnetic field in nav frame
% https://www.ngdc.noaa.gov/geomag/calculators/magcalc.shtml#igrfwmm
%North Comp East Comp Vertical Comp @ 42N 10E
%24,586.8 nT	1,521.2 nT	39,664.7 nT

mag_n = [0.24 0 0.40]'; % approx Gauss field, no declination 

%compute Cnb
Cz=[cos(rpy(3))     sin(rpy(3))     0; ...
    -sin(rpy(3))    cos(rpy(3))     0; ...
    0               0               1];

Cy=[cos(rpy(2))     0               -sin(rpy(2)); ...
    0               1               0; ...
    sin(rpy(2))     0               cos(rpy(2))];

Cx=[1               0               0;...
    0               cos(rpy(1))     sin(rpy(1)); ...
    0               -sin(rpy(1))    cos(rpy(1))];

Cnb = (Cx*Cy*Cz);
mag_b = Cnb*mag_n;

== matlab function navigation_filter_flat_earth_noise/Navigation Filter SINGLE 50 Hz4  ==
  data: flagINITOK input single size=1; flagGPS input single size=1; flagBARO input single size=1; xout output single size=9; measure input single size=9; Q parameter single size=[9,9]; GPS_cov parameter single size=5; BARO_cov parameter single size=1; IMU_cov parameter single size=3; Pout output single
function [xout,Pout] = GPS_BARO_KF_opt( flagINITOK, flagGPS, flagBARO, measure, Q, GPS_cov, BARO_cov, IMU_cov)
%% definition of variables
persistent P %covariance matrix 
persistent x %state vector
persistent filter_running
%filter matrices and constants
persistent A B 
persistent C_GPS_tot R_GPS_tot C_GPS_pos_vel R_GPS_pos_vel C_BARO R_BARO C_IMU R_IMU

if isempty(P)
    P = single(0.1)*Q;
    %initialize state with first measure
    x = single(zeros(9,1));
    
    filter_running = logical(false); %filter starts in OFF, must wait for flagINITOK to become true
    %prepare constant matrices for future use
    dt = single(0.02); 
    %u  = 0;
    subM = [1, dt, 0.5*dt^2;
            0,  1,       dt;
            0,  0,        1];
    A = [subM,zeros(3,3),zeros(3,3);
         zeros(3,3), subM, zeros(3,3);
         zeros(3,3),zeros(3,3),subM];
    B = single(zeros(9,1));
    B(9) = 1;  

    % Covariance state matrix
    % px|vx|ax|py|vy|ay|pz|vz|az
    % Q from mask 

    % Covariance output matrix
    % GPS covariances = px|py|vx|vy|vz
    % GPS_cov  = [0.03, 0.05, 0.016, 0.014, 0.36]; from mask
    % IMU covariances = ax|ay|az
    %IMU_cov  = 1000*[0.07, 0.07, 0.09];    from amsk
    %BARO_cov =  1.7; from amsk 

    %output matrices 
    %tutte le misure disponibili 
    C_GPS_tot = single([ 1 0 0  0 0 0  0 0 0;
                  0 1 0  0 0 0  0 0 0;
                  0 0 1  0 0 0  0 0 0;
                  0 0 0  1 0 0  0 0 0;
                  0 0 0  0 1 0  0 0 0;
                  0 0 0  0 0 1  0 0 0;
                  0 0 0  0 0 0  1 0 0;
                  0 0 0  0 0 0  0 0 1]);
    R_GPS_tot = diag([GPS_cov(1),GPS_cov(3), IMU_cov(1),...
                  GPS_cov(2),GPS_cov(4), IMU_cov(2),...
                  BARO_cov,   IMU_cov(3)]);
    % vel GPS, pos GPS & IMU
    C_GPS_pos_vel = single([ 1 0 0  0 0 0  0 0 0;
                      0 1 0  0 0 0  0 0 0;
                      0 0 1  0 0 0  0 0 0;
                      0 0 0  1 0 0  0 0 0;
                      0 0 0  0 1 0  0 0 0;
                      0 0 0  0 0 1  0 0 0;
                      0 0 0  0 0 0  0 0 1]); 
    R_GPS_pos_vel = diag([GPS_cov(1),GPS_cov(3), IMU_cov(1),...
                          GPS_cov(2),GPS_cov(4), IMU_cov(2),...
                           IMU_cov(3)]);
    % Baro & IMU
    C_BARO = single([0, 0, 1, 0, 0, 0, 0, 0, 0;
              0, 0, 0, 0, 0, 1, 0, 0, 0;
              0, 0, 0, 0, 0, 0, 1, 0, 0
              0, 0, 0, 0, 0, 0, 0, 0, 1]);
    R_BARO = diag([IMU_cov(1),...
                   IMU_cov(2),...
                   BARO_cov, IMU_cov(3)]);
    % solo IMU
    C_IMU = single([0, 0, 1, 0, 0, 0, 0, 0, 0;
             0, 0, 0, 0, 0, 1, 0, 0, 0;
             0, 0, 0, 0, 0, 0, 0, 0, 1]);
    R_IMU = diag([IMU_cov(1),...
                  IMU_cov(2),...
                  IMU_cov(3)]);
    
end

%% initialization 
if and(not(filter_running),flagINITOK),
    % if filter is not running and initialization can be performed 
    % => initialize state = measure
    % => notify filter is running
    x= measure;
    filter_running = true;
end


u  = single(0);


if filter_running, 
    %% select update type (removed fuse types with separate gps pos and vel flags)
    if(flagGPS && flagBARO)
        fuse = 1;
    elseif(flagGPS)
        fuse = 2;
    elseif(flagBARO)
        fuse = 7;
    else
        fuse = 8;
    end

    %% Prediction
    [x, P] = predict(A, B, x, u, Q, P);


    %% Update
    switch fuse
        case 1
            % all measurements
            y = [measure(1), measure(2), measure(3), measure(4), measure(5), ...
                 measure(6), measure(7), measure(9)]';
            [x, P] = update(A, C_GPS_tot, x, y, P, R_GPS_tot);
        case 2
            % measurements of: pos GPS, vel GPS, IMU
            y = [measure(1), measure(2), measure(3), measure(4), measure(5), ...
                 measure(6),  measure(9)]';
            [x, P] = update(A, C_GPS_pos_vel, x, y, P, R_GPS_pos_vel);
        case 7
            % measurements of: BARO, IMU
            y = [measure(3), measure(6), measure(7), measure(9)]';
            [x, P] = update(A, C_BARO, x, y, P, R_BARO);
        case 8
            y = [measure(3), measure(6), measure(9)]';
            [x, P] = update(A, C_IMU, x, y, P, R_IMU);
                     
    end
    
      
end

xout = x;
Pout = P;
end

function [x, P] = predict(A, B, x, u, Q, P)
    x = A*x + B*u;
    P = A*P*A' + Q;
end

function [x, P] = update(A, C, x, y, P, R)
    K = P*C'*inv(R + C*P*C');
    x = x + K*(y - C*x);
    P = (eye(9) - K*C)*P;
    %P = 0.5*(P + transpose(P)); 
end

== matlab function navigation_filter_flat_earth_noise/flat earth POS VEL mechanization/make Cbn ==
  data: rpy input; Cbn output
function Cbn = make_Cbn(rpy)
%compute Cbn
Cz=[cos(rpy(3))     sin(rpy(3))     0; ...
    -sin(rpy(3))    cos(rpy(3))     0; ...
    0               0               1];

Cy=[cos(rpy(2))     0               -sin(rpy(2)); ...
    0               1               0; ...
    sin(rpy(2))     0               cos(rpy(2))];

Cx=[1               0               0;...
    0               cos(rpy(1))     sin(rpy(1)); ...
    0               -sin(rpy(1))    cos(rpy(1))];

Cbn = (Cx*Cy*Cz)';

== matlab function navigation_filter_flat_earth_noise/make Cbn2 ==
  data: rpy input; xyz_n output; xyz_b input
function xyz_n = rot_to_nav(rpy,xyz_b)

%compute Cbn
Cz=[cos(rpy(3))     sin(rpy(3))     0; ...
    -sin(rpy(3))    cos(rpy(3))     0; ...
    0               0               1];

Cy=[cos(rpy(2))     0               -sin(rpy(2)); ...
    0               1               0; ...
    sin(rpy(2))     0               cos(rpy(2))];

Cx=[1               0               0;...
    0               cos(rpy(1))     sin(rpy(1)); ...
    0               -sin(rpy(1))    cos(rpy(1))];

Cbn = (Cx*Cy*Cz)';
xyz_n = Cbn*xyz_b;

== matlab function navigation_filter_flat_earth_noise/Attitude Filter MPU/DCM_MARG_QUAT/dcm_marg ==
  data: euler_out output single; a_ned output single; gyro input single; acc input single; mag input single; q input single; e_int_a input single; e_int_m input single; q_out output single; Kp parameter single; Ki parameter single; T parameter single; e_int_out_a output single; e_int_out_m output single; Rt output; biases output single
function [euler_out, a_ned, q_out, e_int_out_a, e_int_out_m,Rt, biases] = fcn(gyro, acc, mag, q, e_int_a, e_int_m, Kp, Ki, T)
%#codegen

persistent ini;

% mode == 0: mag errors don't affect roll and pitch angles
% mode == 1: standard implementation, roll, pitch and yaw depend on
% acceleroters and magnetos in the same measure
mode = 0;

% Mag and accelerometers MUST have non null norm, if they have null
% norm an error occurred and filter probably will get confused, adjust mag
% and acc values to try to avoid filter problems. 

if (norm(acc) < 1e-4)
    acc = single([0; 0; -9.81]);
end

if (norm(mag) < 1e-4)
    mag = single([0.234; 0.008; 0.404]);
end

% Init quaternion using the first accelerometers and magnetometers reading
% in triad algorithm.

if (isempty(ini))
    q = qtriad(acc, mag);
    ini = 1;
end

q1 = q(1);
q2 = q(2);
q3 = q(3);
q4 = q(4);

gx = gyro(1);
gy = gyro(2);
gz = gyro(3);

ax = acc(1);
ay = acc(2);
az = acc(3);

mx = mag(1);
my = mag(2);
mz = mag(3);

% Rt rotates NED to body, and obviously converts body cordinates into ned
% coordinates.
 
Rt = [1 - 2*q3^2 - 2*q4^2, 2*(q2*q3-q1*q4), 2*(q2*q4+q1*q3);
      2*(q2*q3+q1*q4), 1 - 2*q2^2 - 2*q4^2, 2*(q3*q4-q1*q2);
      2*(q2*q4-q1*q3), 2*(q3*q4+q1*q2), 1 - 2*q2^2 - 2*q3^2];

% Filter implementation
 
h = Rt*[mx; my; mz];

bx = sqrt(h(1)^2+h(2)^2);
bz = abs(h(3));

norm_a = sqrt(ax^2+ay^2+az^2+eps);
e_a = cross([ax ay az]'/norm_a, Rt'*[0 0 -1]');
norm_m = sqrt(mx^2+my^2+mz^2+eps);
norm_b = sqrt(bx^2+bz^2+eps);
e_m = cross([mx my mz]'/norm_m, Rt'*[bx 0 bz]'/norm_b);
e_m = single(zeros(3,1)); %no mag correction
if (mode == 0)
    
    e_int_out_a = e_int_a + T*[e_a(1:2); 0];
    e_int_out_m = e_int_m + T*[0; 0; e_m(3)];
    e_int_out_m = single(zeros(3,1)); 
%     e_m = [0; 0; e_m(3)];
    g = [gx; gy; gz] + Kp*[e_a(1:2); e_m(3)] + Ki*(e_int_out_a + e_int_out_m);

else
    
    e_int_out_a = e_int_a + T*e_a;
    e_int_out_m = e_int_m + T*e_m;
    e_int_out_m = single(zeros(3,1));
%     e_m = [0; 0; e_m(3)];
    g = [gx; gy; gz] + Kp*(e_a + e_m) + Ki*(e_int_out_a + e_int_out_m);
    
end

gx = g(1);
gy = g(2);
gz = g(3);

% Quaternion integration

dq1 = (-q2*gx - q3*gy - q4*gz)/2;
dq2 = (q1*gx + q3*gz - q4*gy)/2;
dq3 = (q1*gy - q2*gz + q4*gx)/2;
dq4 = (q1*gz + q2*gy - q3*gx)/2;

q1 = q1 + dq1*T;
q2 = q2 + dq2*T;
q3 = q3 + dq3*T;
q4 = q4 + dq4*T;

% Quaternion normalization

norm_q = sqrt(q1*q1 + q2*q2 + q3*q3 + q4*q4);
q1 = q1 / norm_q;
q2 = q2 / norm_q;
q3 = q3 / norm_q;
q4 = q4 / norm_q;

q_out = [q1; q2; q3; q4];

% Rt rotates NED to body, and obviously converts body cordinates into ned
% coordinates.

Rt = [1 - 2*q3^2 - 2*q4^2, 2*(q2*q3-q1*q4), 2*(q2*q4+q1*q3);
      2*(q2*q3+q1*q4), 1 - 2*q2^2 - 2*q4^2, 2*(q3*q4-q1*q2);
      2*(q2*q4-q1*q3), 2*(q3*q4+q1*q2), 1 - 2*q2^2 - 2*q3^2];

% Obtain rpy angles
 
psi = atan2(2*(q2*q3+q1*q4), 1 - 2*q3^2 - 2*q4^2);
theta = atan2(-2*(q2*q4-q1*q3), sqrt((2*(q3*q4+q1*q2))^2 + (1 - 2*q2^2 - 2*q3^2)^2));
phi = atan2(2*(q3*q4+q1*q2), 1 - 2*q2^2 - 2*q3^2);

% Compute accelerations in NED

a_ned = Rt*acc;

euler_out = [phi; theta; psi];

% Suppose that mean of integral correction is bias value

biases = -Ki*(e_int_out_a + e_int_out_m);

end

function R = rotz(a)
R = [ cos(a), -sin(a), 0; sin(a), cos(a), 0 ; 0, 0, 1];
end

function R = rotx(a)
R = [ 1, 0, 0; 0, cos(a), -sin(a); 0, sin(a), cos(a);];
end

function R = roty(a)
R = [ cos(a), 0, sin(a) ; 0, 1, 0, ; -sin(a), 0, cos(a)];
end

% Triad algorithm

function q_out = qtriad(acc, mag)

ib = acc/norm(acc);
ir = [0; 0; -1];
mb = mag;
mr = [0.234; 0.008; 0.404];
jb = cross(ib,mb);
jb = jb/norm(jb);
jr = cross(ir,mr);
jr = jr/norm(jr);
kb = cross(ib,jb);
kr = cross(ir,jr);
c = (ib*ir' + jb*jr' + kb*kr')';

q1 = 0.5*sqrt(1+c(1,1)+c(2,2)+c(3,3));
q2 = 0.25/q1*(c(3,2)-c(2,3));
q3 = 0.25/q1*(c(1,3)-c(3,1));
q4 = 0.25/q1*(c(2,1)-c(1,2));

q_out = [q1 q2 q3 q4]';
    
end
